simulink subsystem "extractEsdStats"  (R2020b)
settings: Solver=VariableStepAuto  StartTime=0.0  StopTime=10.0  RelTol=1e-3
settings Model: Creator=trevor  LastModifiedBy=trevor

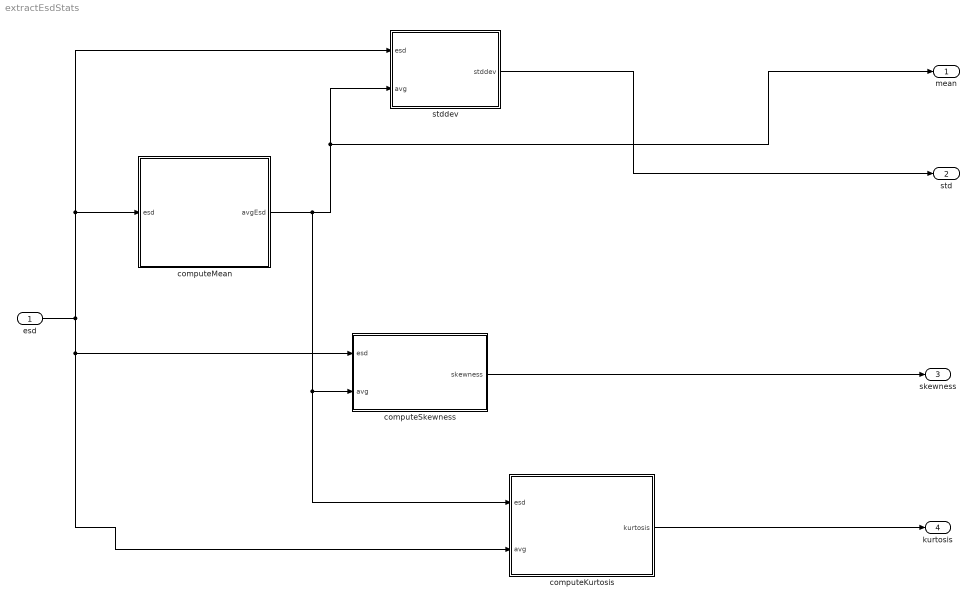
== system extractEsdStats ==
  esd : Inport
  computeKurtosis : Subsystem
  computeMean : Subsystem
  computeSkewness : Subsystem
  stddev : Subsystem
  mean : Outport
  std : Outport  Port=2
  skewness : Outport  Port=3
  kurtosis : Outport  Port=4
  wires:
  stddev/1(stddev) -> std/1
  esd/1 -> stddev/1(esd), computeMean/1(esd), computeSkewness/1(esd), computeKurtosis/2(avg)
  computeKurtosis/1(kurtosis) -> kurtosis/1
  computeSkewness/1(skewness) -> skewness/1
  computeMean/1(avgEsd) -> stddev/2(avg), mean/1, computeKurtosis/1(esd), computeSkewness/2(avg)

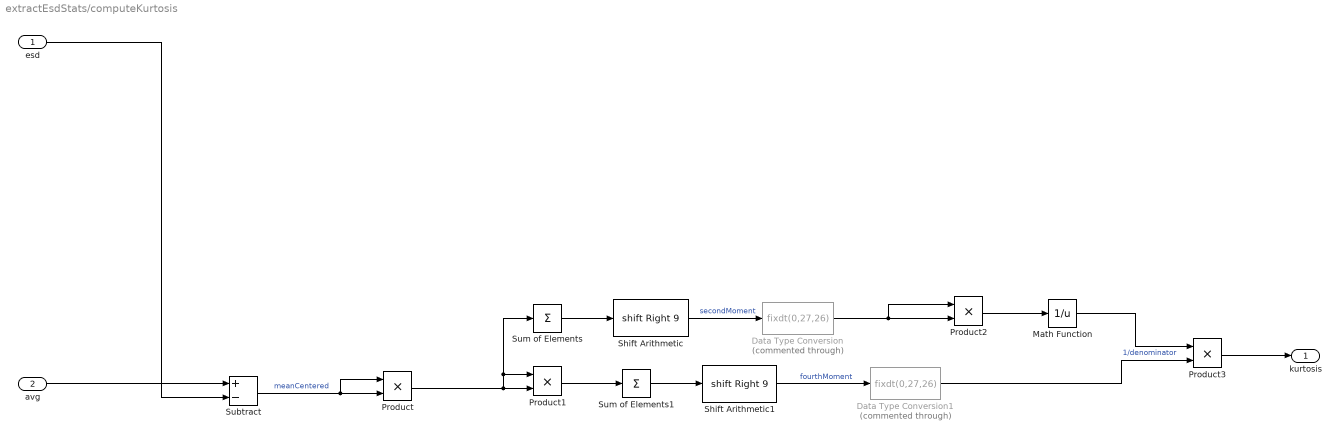
== system extractEsdStats/computeKurtosis ==
  esd : Inport
  avg : Inport  Port=2
  Data Type Conversion : DataTypeConversion  Commented=through  OutDataTypeStr=fixdt(0,27,26)
  Data Type Conversion1 : DataTypeConversion  Commented=through  OutDataTypeStr=fixdt(0,27,26)
  Math Function : Math  Operator=reciprocal  RndMeth=Zero  SaturateOnIntegerOverflow=on  OutDataTypeStr=Inherit: Inherit via internal rule
  Product : Product
  Product1 : Product  OutDataTypeStr=Inherit: Same as first input
  Product2 : Product  OutDataTypeStr=Inherit: Same as first input
  Product3 : Product  OutDataTypeStr=Inherit: Match scaling
  Shift Arithmetic : ArithShift  BitShiftNumber=9  BitShiftDirection=Right
  Shift Arithmetic1 : ArithShift  BitShiftNumber=9  BitShiftDirection=Right
  Subtract : Sum  Inputs=+-
  Sum of Elements : Sum  Inputs=+
  Sum of Elements1 : Sum  Inputs=+
  kurtosis : Outport
  wires:
  Data Type Conversion1/1 -> Product3/2
  Data Type Conversion/1 -> Product2/2, Product2/1
  Math Function/1 -> Product3/1  "1/denominator"
  Sum of Elements/1 -> Shift Arithmetic/1
  Product/1 -> Product1/2, Product1/1, Sum of Elements/1
  Sum of Elements1/1 -> Shift Arithmetic1/1
  Shift Arithmetic/1 -> Data Type Conversion/1  "secondMoment"
  avg/1 -> Subtract/1
  esd/1 -> Subtract/2
  Product3/1 -> kurtosis/1
  Product1/1 -> Sum of Elements1/1
  Subtract/1 -> Product/2, Product/1  "meanCentered"
  Shift Arithmetic1/1 -> Data Type Conversion1/1  "fourthMoment"
  Product2/1 -> Math Function/1

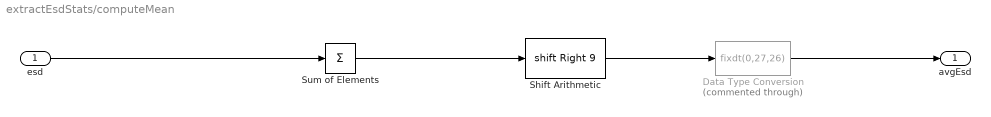
== system extractEsdStats/computeMean ==
  esd : Inport
  Data Type Conversion : DataTypeConversion  Commented=through  OutDataTypeStr=fixdt(0,27,26)
  Shift Arithmetic : ArithShift  BitShiftNumber=9  BitShiftDirection=Right
  Sum of Elements : Sum  Inputs=+
  avgEsd : Outport
  wires:
  Data Type Conversion/1 -> avgEsd/1
  Sum of Elements/1 -> Shift Arithmetic/1
  esd/1 -> Sum of Elements/1
  Shift Arithmetic/1 -> Data Type Conversion/1

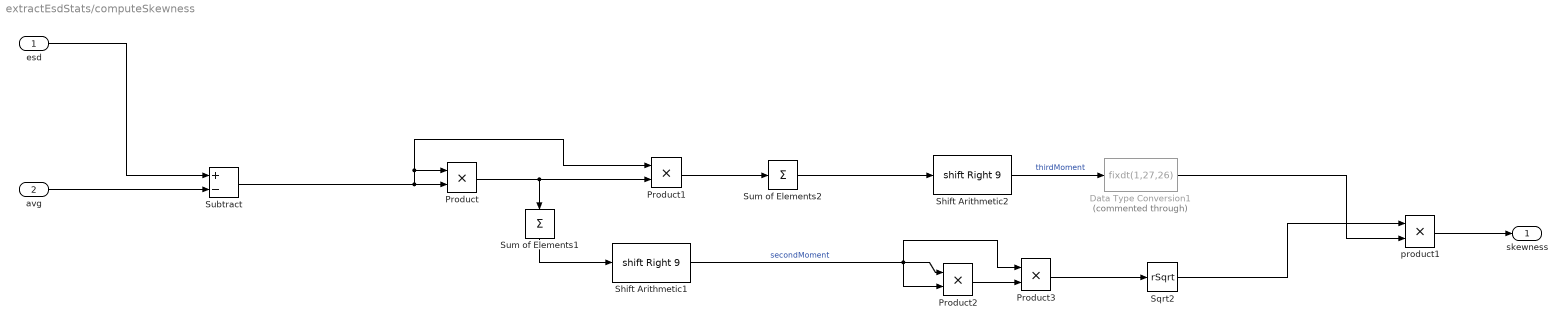
== system extractEsdStats/computeSkewness ==
  esd : Inport
  avg : Inport  Port=2
  Data Type Conversion1 : DataTypeConversion  Commented=through  OutDataTypeStr=fixdt(1,27,26)
  Product : Product  OutMin=0  OutMax=1
  Product1 : Product  OutDataTypeStr=Inherit: Same as first input
  Product2 : Product  OutDataTypeStr=Inherit: Same as first input
  Product3 : Product  OutDataTypeStr=Inherit: Same as first input
  Shift Arithmetic1 : ArithShift  BitShiftNumber=9  BitShiftDirection=Right
  Shift Arithmetic2 : ArithShift  BitShiftNumber=9  BitShiftDirection=Right
  Sqrt2 : Sqrt  Operator=rSqrt  Iterations=10  SaturateOnIntegerOverflow=on  OutDataTypeStr=Inherit: Inherit via internal rule
  Subtract : Sum  Inputs=+-
  Sum of Elements1 : Sum  Inputs=+
  Sum of Elements2 : Sum  Inputs=+
  product1 : Product  Inputs=**  RndMeth=Zero  SaturateOnIntegerOverflow=on
  skewness : Outport
  wires:
  Product2/1 -> Product3/2
  Product3/1 -> Sqrt2/1
  Data Type Conversion1/1 -> product1/2
  Sqrt2/1 -> product1/1
  Subtract/1 -> Product/2, Product/1, Product1/1
  Sum of Elements2/1 -> Shift Arithmetic2/1
  Sum of Elements1/1 -> Shift Arithmetic1/1
  product1/1 -> skewness/1
  Shift Arithmetic2/1 -> Data Type Conversion1/1  "thirdMoment"
  Shift Arithmetic1/1 -> Product2/1, Product3/1, Product2/2  "secondMoment"
  Product1/1 -> Sum of Elements2/1
  Product/1 -> Product1/2, Sum of Elements1/1
  avg/1 -> Subtract/2
  esd/1 -> Subtract/1

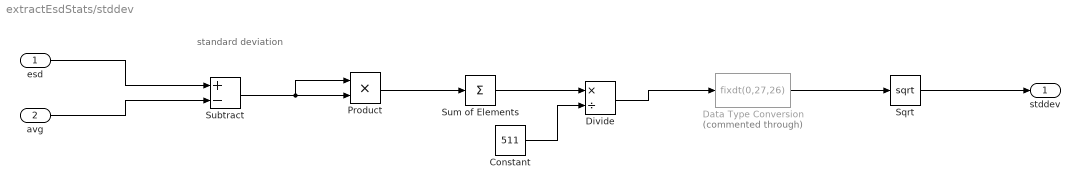
== system extractEsdStats/stddev ==
  note: standard deviation
  esd : Inport
  avg : Inport  Port=2
  Constant : Constant  Value=511  OutDataTypeStr=Inherit: Inherit via back propagation  SampleTime=-1
  Data Type Conversion : DataTypeConversion  Commented=through  OutDataTypeStr=fixdt(0,27,26)
  Divide : Product  Inputs=*/  RndMeth=Zero  SaturateOnIntegerOverflow=on
  Product : Product
  Sqrt : Sqrt  SaturateOnIntegerOverflow=on
  Subtract : Sum  Inputs=+-  OutDataTypeStr=Inherit: Same as accumulator
  Sum of Elements : Sum  Inputs=+
  stddev : Outport
  wires:
  Constant/1 -> Divide/2
  Sum of Elements/1 -> Divide/1
  esd/1 -> Subtract/1
  Sqrt/1 -> stddev/1
  Subtract/1 -> Product/2, Product/1
  avg/1 -> Subtract/2
  Divide/1 -> Data Type Conversion/1
  Product/1 -> Sum of Elements/1
  Data Type Conversion/1 -> Sqrt/1
